simulink model "threedoftest"  (R2015b)
settings: Solver=VariableStepAuto  StartTime=0.0  StopTime=10.0  RelTol=1e-3
libraries: aerolib3dof2 x1
settings Model: Creator=Jamie  LastModifiedBy=Jamie

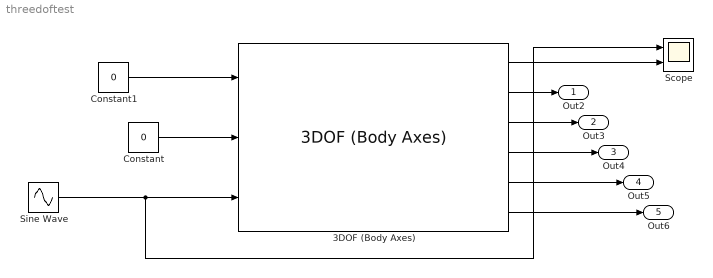
== system threedoftest ==
  3DOF (Body Axes) : aerolib3dof2/3DOF (Body Axes)  units=Metric (MKS)  mtype=Fixed  v_ini=100  theta_ini=0  alpha_ini=0  q_ini=0  pos_ini=[0 0]  mass=1.0  mass_e=0.5  mass_f=3.0  Iyy=1.0  Iyy_e=0.5  Iyy_f=3.0  g_in=Internal  g=9.81  vre_flag=on
  Constant : Constant  Value=0
  Constant1 : Constant  Value=0
  Scope : Scope  NumInputPorts=2
  Sine Wave : Sin  SampleTime=0
  Out2 : Outport
  Out3 : Outport  Port=2
  Out4 : Outport  Port=3
  Out5 : Outport  Port=4
  Out6 : Outport  Port=5
  wires:
  Constant/1 -> 3DOF (Body Axes)/2
  3DOF (Body Axes)/2 -> Out2/1
  3DOF (Body Axes)/3 -> Out3/1
  3DOF (Body Axes)/4 -> Out4/1
  3DOF (Body Axes)/5 -> Out5/1
  3DOF (Body Axes)/6 -> Out6/1
  Constant1/1 -> 3DOF (Body Axes)/1
  3DOF (Body Axes)/1 -> Scope/2
  Sine Wave/1 -> Scope/1, 3DOF (Body Axes)/3
